simulink library "resolveDotPos_ul"  (R2018b)
settings: Solver=VariableStepAuto  StartTime=0.0  StopTime=10.0  RelTol=1e-3
settings Model: Creator=MAE-NCSUCORE  LastModifiedBy=MAE-NCSUCORE

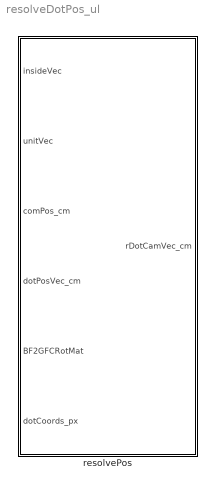
== system resolveDotPos_ul ==
  resolvePos : Subsystem

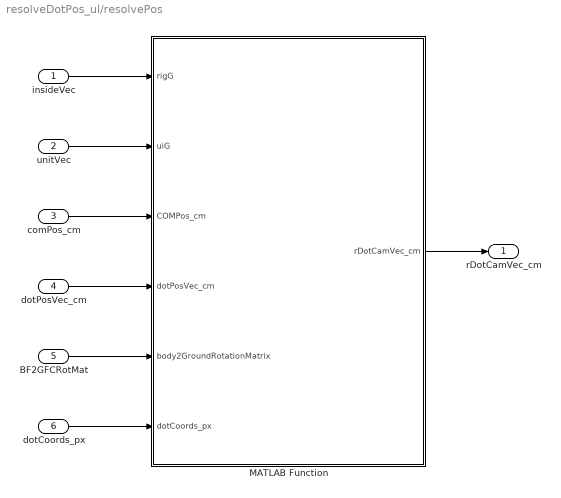
== system resolveDotPos_ul/resolvePos ==
  insideVec : Inport
  unitVec : Inport  Port=2
  comPos_cm : Inport  Port=3
  dotPosVec_cm : Inport  Port=4
  BF2GFCRotMat : Inport  Port=5
  dotCoords_px : Inport  Port=6
  MATLAB Function : MATLAB Function  TreatAsAtomicUnit=on
  rDotCamVec_cm : Outport
  wires:
  MATLAB Function/1(rDotCamVec_cm) -> rDotCamVec_cm/1
  insideVec/1 -> MATLAB Function/1(rigG)
  comPos_cm/1 -> MATLAB Function/3(COMPos_cm)
  BF2GFCRotMat/1 -> MATLAB Function/5(body2GroundRotationMatrix)
  unitVec/1 -> MATLAB Function/2(uiG)
  dotCoords_px/1 -> MATLAB Function/6(dotCoords_px)
  dotPosVec_cm/1 -> MATLAB Function/4(dotPosVec_cm)

== matlab function resolveDotPos_ul/resolvePos/MATLAB Function ==
  data: rigG input; rDotCamVec_cm output; uiG input; COMPos_cm input; dotPosVec_cm input; body2GroundRotationMatrix input; dotCoords_px input
function rDotCamVec_cm  = resolveDotPos(rigG,uiG,COMPos_cm,dotPosVec_cm,...
    body2GroundRotationMatrix,dotCoords_px)

[rDotCamVec_cm] = resolveDotPos(rigG,uiG,COMPos_cm,dotPosVec_cm,...
    body2GroundRotationMatrix,dotCoords_px);
